simulink subsystem "PvtSubSys_LONC"  (R2020b)
settings: Solver=VariableStepAuto  StartTime=0.0  StopTime=10.0  RelTol=1e-3
undefined symbols (not defined in the file): P_Global_TireRadius_m, P_Global_Weight_N, P_LongCtrl_AxvRoadSlopeThrd, P_LongCtrl_SlideFlagEnable, P_LongCtrl_TotWheelTrqRatio, P_LongCtrl_VLC_fRollCoef, P_LongCtrl_VLC_WindArea, P_LongCtrl_VLCaccelMinHoldXAxis, P_LongCtrl_VLCaccelMinHoldYAxis, P_LongCtrl_VLCaccelMinSlidHoldXAxis, P_LongCtrl_VLCaccelMinSlidHoldYAxis, P_LongCtrl_VLCaDiffCharCoefKiEnableXAxis, P_LongCtrl_VLCaDiffCharCoefKiXAxis, P_LongCtrl_VLCaDtThresUpdateTorq, P_LongCtrl_VLCaXCDeadZoneProp_Y, P_LongCtrl_VLCaxCtrlDevDeadZoneChar_Y, P_LongCtrl_VLCaxCtrlDevEC2DCMax, P_LongCtrl_VLCaxCtrlDevFastQuitDCMode, P_LongCtrl_VLCaxCtrlDevThresAddEC2DCCharYAxis, P_LongCtrl_VLCaxCtrlDevTresAddDC2ECYAxis, P_LongCtrl_VLCaxDtCharAxCtrlDevTresAddDC2ECXAxis, P_LongCtrl_VLCaxDtCharAxCtrlDevTresAddEC2DCXAxis, P_LongCtrl_VLCAxTarDtThreEnableI, P_LongCtrl_VLCaxvRoadSlopeDC4CharXAxis, P_LongCtrl_VLCaxvRoadSlopeDC4CharYAxis, P_LongCtrl_VLCAxvTracMinDC1FullFillXAxis, P_LongCtrl_VLCAxvTracMinDC1FullFillYAxis, P_LongCtrl_VLCcoefFXAxis, P_LongCtrl_VLCcoefFYAxis, P_LongCtrl_VLCcoefIFadeOut1Calc, P_LongCtrl_VLCcoefIFadeOut1Condition, P_LongCtrl_VLCcoefIFadeOut2Calc, P_LongCtrl_VLCcoefIFadeOut2Condition, P_LongCtrl_VLCcoefIFadeOut3Calc, P_LongCtrl_VLCcoefIFadeOut3Condition, P_LongCtrl_VLCcoefKiDiffDtEnlargeYAxis, P_LongCtrl_VLCcoefKiEnableYAxis, P_LongCtrl_VLCcoefKiEnlargeADiffYAxis, P_LongCtrl_VLCcoefPIYAxis, P_LongCtrl_VLCCounterAxvTracMinTimeout, P_LongCtrl_VLCCounterDC2ECTorqDelay, P_LongCtrl_VLCCounterDrvOff2EC, P_LongCtrl_VLCdaxTarEC2DCMax, P_LongCtrl_VLCdiffDtCharCoefKiEnlargeXAxis, P_LongCtrl_VLCdriveOffAxUpLimXAxix, P_LongCtrl_VLCdriveOffAxUpLimYAxix, P_LongCtrl_VLCDtAxvRef2UpperBandDC5, P_LongCtrl_VLCengEfficientCharYAxis, P_LongCtrl_VLCengInverseEfficientYAxis, P_LongCtrl_VLCIACompensionNeg, P_LongCtrl_VLCIACompensionPos, P_LongCtrl_VLCjerkHoldXAxis, P_LongCtrl_VLCjerkHoldYAxis, P_LongCtrl_VLCjerkSlidHoldXAxis, P_LongCtrl_VLCjerkSlidHoldYAxis, P_LongCtrl_VLCki, P_LongCtrl_VLCkp, P_LongCtrl_VLCks, P_LongCtrl_VLCLowerJerkCounterDrvOff2EC, P_LongCtrl_VLCMaRatioCharMaYAxis ... (+12)
libraries: simulink x34
(part 1 of 3)
settings Model: Creator=GW00133806  LastModifiedBy=GW00201118

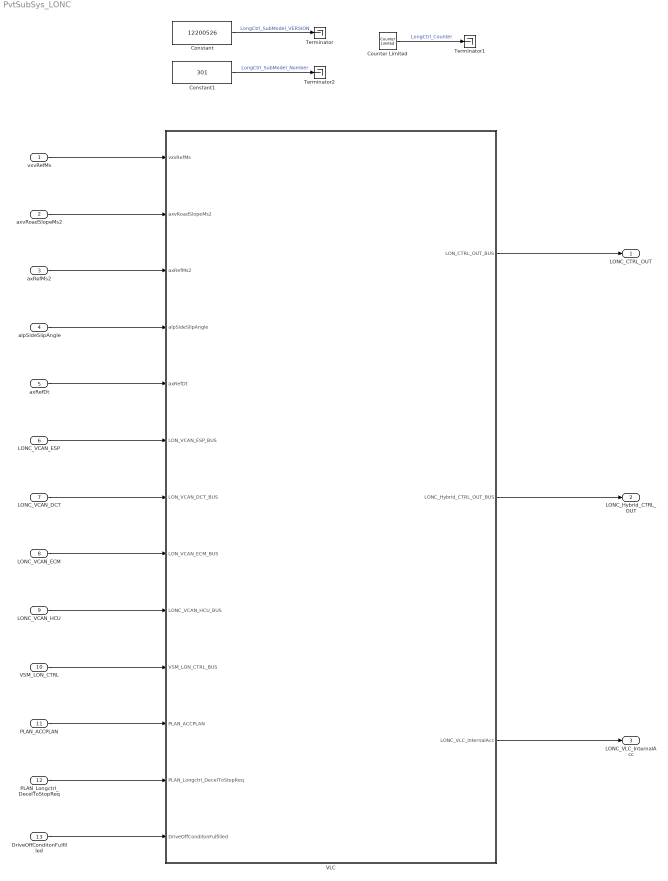
== system PvtSubSys_LONC ==
  vxvRefMs : Inport  Description=m/s | 车速  OutDataTypeStr=single  PortDimensions=1  BusOutputAsStruct=on
  axvRoadSlopeMs2 : Inport  Description=m/s^2 | 坡道加速度  Port=2  OutDataTypeStr=single  PortDimensions=1  BusOutputAsStruct=on
  axRefMs2 : Inport  Description=m/s^2 | 自车参考加速度  Port=3  OutDataTypeStr=single  PortDimensions=1  BusOutputAsStruct=on
  alpSideSlipAngle : Inport  Description=rad | 后轮侧滑角  Port=4  OutDataTypeStr=single  PortDimensions=1  BusOutputAsStruct=on
  axRefDt : Inport  Description=m/s^3 | 加速度变化率  Port=5  OutDataTypeStr=single  PortDimensions=1  BusOutputAsStruct=on
  LONC_VCAN_ESP : Inport  Description=|  Port=6  OutDataTypeStr=Bus: VCAN_ESP_MSG_BUS  PortDimensions=1  BusOutputAsStruct=on
      | NoBrkForce          是否存在轮缸压力
      | VehStandstill       判断车辆是否静止
  LONC_VCAN_DCT : Inport  Description="SHIFT_IN_PROGRESS    换挡进行中"  Port=7  OutDataTypeStr=Bus: VCAN_DCT_MSG_BUS  PortDimensions=1  BusOutputAsStruct=on
  LONC_VCAN_ECM : Inport  Description=|  Port=8  OutDataTypeStr=Bus: VCAN_ECM_MSG_BUS  PortDimensions=1  BusOutputAsStruct=on
      | NetEngTrq               当前实际扭矩
      | MaxEngTrqNorm           最大扭矩
      | EngTrqMinAct            最小可执行扭矩
      | EngTrqMaxActSpd
      | EngSpd                  发动机转速
  LONC_VCAN_HCU : Inport  Port=9  OutDataTypeStr=Bus: VCAN_HCU_MSG_BUS  PortDimensions=1  BusOutputAsStruct=on
  VSM_LON_CTRL : Inport  Description=|  Port=10  OutDataTypeStr=Bus: VSM_LON_CTRL_BUS  PortDimensions=1  BusOutputAsStruct=on
      | ACCSts              ACC状态
      | ACC_DrvOffReq       起步标志位
  PLAN_ACCPLAN : Inport  Description=|  Port=11  OutDataTypeStr=Bus: PLAN_ACCPLAN_BUS
      | ACC_axvCvAim                         期望加速度
      | ACC_axv_ComfortBandLowerValue        期望加速度下限
      | ACC_axv_ComfortBandUpperValue        期望加速度上限
      | ACC_DecelerateJerk                   加速度变化率下限
      | ACC_AccelerateJerk                   加速度变化率上限
      | ACC_BrakePrefer                      制动优先标志位
  PLAN_Longctrl_DecelToStopReq : Inport  Description=boolean | 制动到停状态  Port=12  OutDataTypeStr=boolean  PortDimensions=1  BusOutputAsStruct=on
  DriveOffConditonFulfilled : Inport  Port=13
  Constant : Constant  Value=12200526  OutDataTypeStr=uint32
  Constant1 : Constant  Value=301  OutDataTypeStr=uint32
  Counter Limited : simulink/Sources/Counter Limited  uplimit=15  tsamp=-1
  Terminator : Terminator
  Terminator1 : Terminator
  Terminator2 : Terminator
  VLC : Subsystem
  LONC_CTRL_OUT : Outport  OutDataTypeStr=Bus: LONC_CTRL_OUT_BUS  PortDimensions=1  BusOutputAsStruct=on
  LONC_Hybrid_CTRL_OUT : Outport  Port=2  OutDataTypeStr=Bus: LONC_Hybrid_CTRL_OUT_BUS  PortDimensions=1  BusOutputAsStruct=on
  LONC_VLC_InternalAcc : Outport  Port=3  OutDataTypeStr=single
  wires:
  vxvRefMs/1 -> VLC/1(vxvRefMs)
  LONC_VCAN_ECM/1 -> VLC/8(LON_VCAN_ECM_BUS)
  Counter Limited/1 -> Terminator1/1  "LongCtrl_Counter"
  Constant/1 -> Terminator/1  "LongCtrl_SubModel_VERSION"
  DriveOffConditonFulfilled/1 -> VLC/13(DriveOffConditonFulfilled)
  VSM_LON_CTRL/1 -> VLC/10(VSM_LON_CTRL_BUS)
  axRefMs2/1 -> VLC/3(axRefMs2)
  alpSideSlipAngle/1 -> VLC/4(alpSideSlipAngle)
  PLAN_Longctrl_DecelToStopReq/1 -> VLC/12(PLAN_Longctrl_DecelToStopReq)
  LONC_VCAN_DCT/1 -> VLC/7(LON_VCAN_DCT_BUS)
  axvRoadSlopeMs2/1 -> VLC/2(axvRoadSlopeMs2)
  VLC/3(LONC_VLC_InternalAcc) -> LONC_VLC_InternalAcc/1
  axRefDt/1 -> VLC/5(axRefDt)
  LONC_VCAN_HCU/1 -> VLC/9(LONC_VCAN_HCU_BUS)
  VLC/1(LON_CTRL_OUT_BUS) -> LONC_CTRL_OUT/1
  PLAN_ACCPLAN/1 -> VLC/11(PLAN_ACCPLAN)
  LONC_VCAN_ESP/1 -> VLC/6(LON_VCAN_ESP_BUS)
  Constant1/1 -> Terminator2/1  "LongCtrl_SubModel_Number"
  VLC/2(LONC_Hybrid_CTRL_OUT_BUS) -> LONC_Hybrid_CTRL_OUT/1

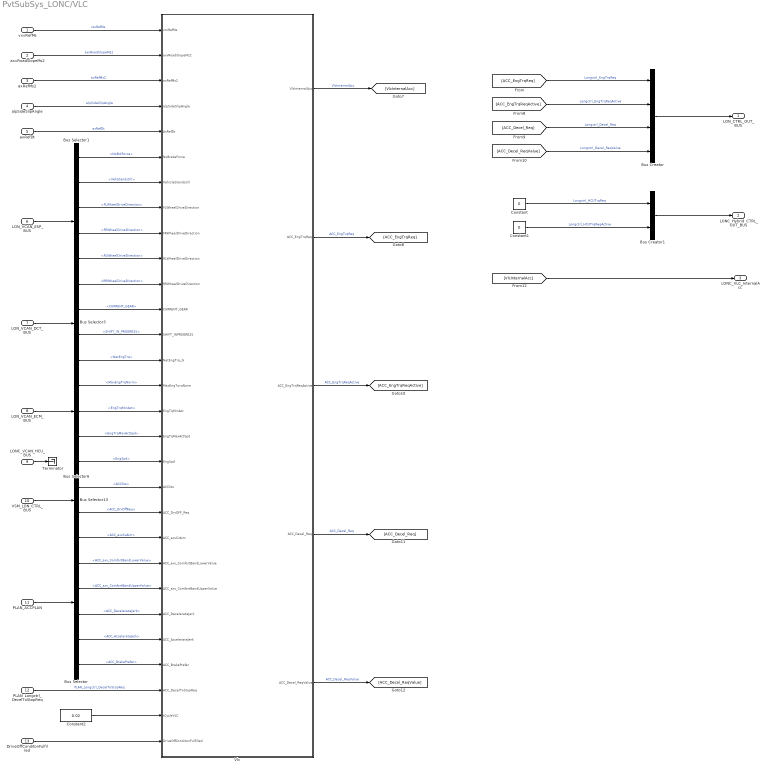
== system PvtSubSys_LONC/VLC ==
  vxvRefMs : Inport
  axvRoadSlopeMs2 : Inport  Port=2
  axRefMs2 : Inport  Port=3
  alpSideSlipAngle : Inport  Port=4
  axRefDt : Inport  Port=5
  LON_VCAN_ESP_BUS : Inport  Port=6  OutDataTypeStr=Bus: VCAN_ESP_MSG_BUS
  LON_VCAN_DCT_BUS : Inport  Port=7  OutDataTypeStr=Bus: VCAN_DCT_MSG_BUS
  LON_VCAN_ECM_BUS : Inport  Port=8  OutDataTypeStr=Bus: VCAN_ECM_MSG_BUS
  LONC_VCAN_HCU_BUS : Inport  Port=9  OutDataTypeStr=Bus: VCAN_HCU_MSG_BUS
  VSM_LON_CTRL_BUS : Inport  Port=10  OutDataTypeStr=Bus: VSM_LON_CTRL_BUS
  PLAN_ACCPLAN : Inport  Port=11  OutDataTypeStr=Bus: PLAN_ACCPLAN_BUS
  PLAN_Longctrl_DecelToStopReq : Inport  Port=12  OutDataTypeStr=boolean
  DriveOffConditonFulfilled : Inport  Port=13
  Bus Creator : BusCreator  Inputs=4  OutDataTypeStr=Bus: LONC_CTRL_OUT_BUS  NonVirtualBus=on
  Bus Creator1 : BusCreator  Inputs=2  OutDataTypeStr=Bus: LONC_Hybrid_CTRL_OUT_BUS  NonVirtualBus=on
  Bus Selector : BusSelector  OutputSignals=ACC_axvCvAim,ACC_axv_ComfortBandLowerValue,ACC_axv_ComfortBandUpperValue,ACC_DecelerateJerk,ACC_AccelerateJerk,ACC_BrakePrefer
  Bus Selector1 : BusSelector  OutputSignals=NoBrkForce,VehStandstill,FLWheelDriveDirection,FRWheelDriveDirection,RLWheelDriveDirection,RRWheelDriveDirection
  Bus Selector13 : BusSelector  OutputSignals=ACCSts,ACC_DrvOffReq
  Bus Selector3 : BusSelector  OutputSignals=CURRENT_GEAR,SHIFT_IN_PROGRESS
  Bus Selector6 : BusSelector  OutputSignals=NetEngTrq,MaxEngTrqNorm,EngTrqMinAct,EngTrqMaxActSpd,EngSpd
  Constant : Constant  Value=0  OutDataTypeStr=single
  Constant1 : Constant  Value=0  OutDataTypeStr=boolean
  Constant2 : Constant  Value=0.02  OutDataTypeStr=single
  Terminator : Terminator
  Vlc : Subsystem  TreatAsAtomicUnit=on
  LON_CTRL_OUT_BUS : Outport  OutDataTypeStr=Bus: LONC_CTRL_OUT_BUS
  LONC_Hybrid_CTRL_OUT_BUS : Outport  Port=2  OutDataTypeStr=Bus: LONC_Hybrid_CTRL_OUT_BUS
  LONC_VLC_InternalAcc : Outport  Port=3  OutDataTypeStr=single
  wires:
  LONC_VCAN_HCU_BUS/1 -> Terminator/1
  Constant/1 -> Bus Creator1/1  "Longctrl_HCUTrqReq"
  Constant1/1 -> Bus Creator1/2  "Longctrl_HCUTrqReqActive"
  Bus Creator1/1 -> LONC_Hybrid_CTRL_OUT_BUS/1
  PLAN_Longctrl_DecelToStopReq/1 -> Vlc/27(ACC_DecelToStopReq)  "PLAN_Longctrl_DecelToStopReq"
  [VlcInternalAcc] -> LONC_VLC_InternalAcc/1
  Bus Selector/1 -> Vlc/21(ACC_axvCvAim)  "<ACC_axvCvAim>"
  Bus Selector/6 -> Vlc/26(ACC_BrakePrefer)  "<ACC_BrakePrefer>"
  Bus Selector/2 -> Vlc/22(ACC_axv_ComfortBandLowerValue)  "<ACC_axv_ComfortBandLowerValue>"
  Bus Selector/3 -> Vlc/23(ACC_axv_ComfortBandUpperValue)  "<ACC_axv_ComfortBandUpperValue>"
  Bus Selector/5 -> Vlc/25(ACC_AccelerateJerk)  "<ACC_AccelerateJerk>"
  Bus Selector/4 -> Vlc/24(ACC_DecelerateJerk)  "<ACC_DecelerateJerk>"
  PLAN_ACCPLAN/1 -> Bus Selector/1
  alpSideSlipAngle/1 -> Vlc/4(alpSideSlipAngle)  "alpSideSlipAngle"
  Bus Selector13/2 -> Vlc/20(ACC_DrvOFF_Req)  "<ACC_DrvOffReq>"
  Bus Selector13/1 -> Vlc/19(ACCSts)  "<ACCSts>"
  VSM_LON_CTRL_BUS/1 -> Bus Selector13/1
  Bus Selector6/5 -> Vlc/18(EngSpd)  "<EngSpd>"
  Bus Selector6/4 -> Vlc/17(EngTqMaxActSpd)  "<EngTrqMaxActSpd>"
  Bus Selector6/3 -> Vlc/16(EngTqMinAct)  "<EngTrqMinAct>"
  Bus Selector6/2 -> Vlc/15(MaxEngTorqNorm)  "<MaxEngTrqNorm>"
  Bus Selector6/1 -> Vlc/14(NetEngTrq_G)  "<NetEngTrq>"
  LON_VCAN_ECM_BUS/1 -> Bus Selector6/1
  LON_VCAN_DCT_BUS/1 -> Bus Selector3/1
  Bus Selector3/2 -> Vlc/13(SHIFT_INPROGRESS)  "<SHIFT_IN_PROGRESS>"
  Bus Selector3/1 -> Vlc/12(CURRENT_GEAR)  "<CURRENT_GEAR>"
  LON_VCAN_ESP_BUS/1 -> Bus Selector1/1
  Bus Selector1/2 -> Vlc/7(VehicleStandstill)  "<VehStandstill>"
  Bus Selector1/1 -> Vlc/6(NoBrakeForce)  "<NoBrkForce>"
  axRefDt/1 -> Vlc/5(AxRefDt)  "axRefDt"
  axRefMs2/1 -> Vlc/3(axRefMs2)  "axRefMs2"
  axvRoadSlopeMs2/1 -> Vlc/2(axvRoadSlopeMs2)  "axvRoadSlopeMs2"
  vxvRefMs/1 -> Vlc/1(vxvRefMs)  "vxvRefMs"
  [ACC_EngTrqReqActive] -> Bus Creator/2  "Longctrl_EngTrqReqActive"
  Vlc/2(ACC_EngTrqReq) -> [ACC_EngTrqReq]  "ACC_EngTrqReq"
  Vlc/4(ACC_Decel_Req) -> [ACC_Decel_Req]  "ACC_Decel_Req"
  Vlc/1(VlcInternalAcc) -> [VlcInternalAcc]  "VlcInternalAcc"
  Vlc/5(ACC_Decel_ReqValue) -> [ACC_Decel_ReqValue]  "ACC_Decel_ReqValue"
  Vlc/3(ACC_EngTrqReqActive) -> [ACC_EngTrqReqActive]  "ACC_EngTrqReqActive"
  Bus Creator/1 -> LON_CTRL_OUT_BUS/1
  [ACC_Decel_Req] -> Bus Creator/3  "Longctrl_Decel_Req"
  [ACC_Decel_ReqValue] -> Bus Creator/4  "Longctrl_Decel_ReqValue"
  [ACC_EngTrqReq] -> Bus Creator/1  "Longctrl_EngTrqReq"
  Constant2/1 -> Vlc/28(tCycleVLC)
  DriveOffConditonFulfilled/1 -> Vlc/29(DriveOffConditonFulfilled)
  Bus Selector1/3 -> Vlc/8(FLWheelDriveDirection)  "<FLWheelDriveDirection>"
  Bus Selector1/4 -> Vlc/9(FRWheelDriveDirection)  "<FRWheelDriveDirection>"
  Bus Selector1/5 -> Vlc/10(RLWheelDriveDirection)  "<RLWheelDriveDirection>"
  Bus Selector1/6 -> Vlc/11(RRWheelDriveDirection)  "<RRWheelDriveDirection>"

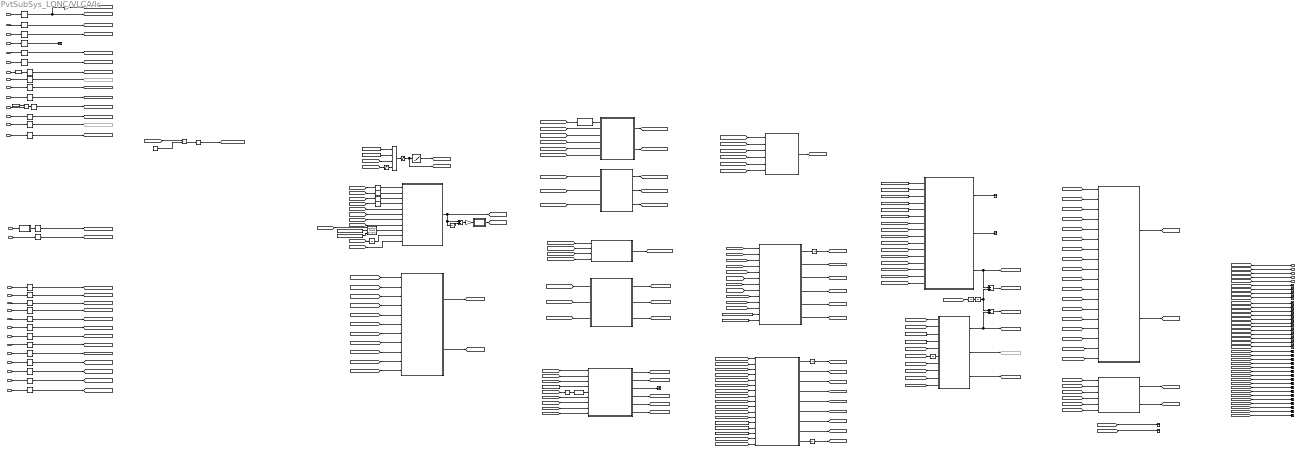
== system PvtSubSys_LONC/VLC/Vlc ==
  vxvRefMs : Inport  OutDataTypeStr=single
  axvRoadSlopeMs2 : Inport  Port=2  OutDataTypeStr=single
  axRefMs2 : Inport  Port=3  OutDataTypeStr=single
  alpSideSlipAngle : Inport  Port=4  OutDataTypeStr=single
  AxRefDt : Inport  Port=5  OutDataTypeStr=single
  NoBrakeForce : Inport  Port=6  OutDataTypeStr=boolean
  VehicleStandstill : Inport  Port=7  OutDataTypeStr=uint8
  FLWheelDriveDirection : Inport  Port=8
  FRWheelDriveDirection : Inport  Port=9
  RLWheelDriveDirection : Inport  Port=10
  RRWheelDriveDirection : Inport  Port=11
  CURRENT_GEAR : Inport  Port=12  OutDataTypeStr=uint8
  SHIFT_INPROGRESS : Inport  Port=13  OutDataTypeStr=boolean
  NetEngTrq_G : Inport  Port=14  OutDataTypeStr=single
  MaxEngTorqNorm : Inport  Port=15  OutDataTypeStr=uint16
  EngTqMinAct : Inport  Port=16  OutDataTypeStr=single
  EngTqMaxActSpd : Inport  Port=17  OutDataTypeStr=single
  EngSpd : Inport  Port=18  OutDataTypeStr=single
  ACCSts : Inport  Port=19  OutDataTypeStr=uint8
  ACC_DrvOFF_Req : Inport  Port=20  OutDataTypeStr=boolean
  ACC_axvCvAim : Inport  Port=21
  ACC_axv_ComfortBandLowerValue : Inport  Port=22
  ACC_axv_ComfortBandUpperValue : Inport  Port=23
  ACC_DecelerateJerk : Inport  Port=24
  ACC_AccelerateJerk : Inport  Port=25
  ACC_BrakePrefer : Inport  Port=26
  ACC_DecelToStopReq : Inport  Port=27
  tCycleVLC : Inport  Port=28
  DriveOffConditonFulfilled : Inport  Port=29
  AxTarUplimit : simulink/Lookup Tables/Lookup Table Dynamic  LookUpMeth=Interpolation-Use End Values  OutDataType=fixdt('single')  OutScaling=[]  OutputDataTypeScalingMode=Specify via dialog  OutDataTypeStr=single  DoSatur=off
  Compare To Constant8 : simulink/Logic and Bit Operations/Compare To Constant  relop===  const=1  OutDataTypeStr=boolean
  Compare To Zero : simulink/Logic and Bit Operations/Compare To Zero  relop===  OutDataTypeStr=boolean
  Constant : Constant  OutDataTypeStr=single
  Constant1 : Constant  Description="1.5         1.5         1.6         1.8           2"  Value=P_LongCtrl_VLCdriveOffAxUpLimYAxix  OutDataTypeStr=single
      settings: AttributesFormatString=%<Description>
  Constant10 : Constant  Description=0.7  Value=P_LongCtrl_VLCaxCtrlDevFastQuitDCMode  OutDataTypeStr=single
      settings: AttributesFormatString=%<Description>
  Constant11 : Constant  Description="0.1         0.1        0.15         0.2         0.2"  Value=P_LongCtrl_VLCaxCtrlDevThresAddEC2DCCharYAxis  OutDataTypeStr=single
      settings: AttributesFormatString=%<Description>
  Constant12 : Constant  Description=0.5  Value=P_LongCtrl_VLCaxCtrlDevEC2DCMax  OutDataTypeStr=single
      settings: AttributesFormatString=%<Description>
  Constant13 : Constant  Description=-0.2  Value=P_LongCtrl_VLCdaxTarEC2DCMax  OutDataTypeStr=single
      settings: AttributesFormatString=%<Description>
  Constant2 : Constant  Description=4  Value=P_LongCtrl_VLCkp  OutDataTypeStr=single
      settings: AttributesFormatString=%<Description>
  Constant3 : Constant  Description="0         0.5           1         1.5           3"  Value=P_LongCtrl_VLCdriveOffAxUpLimXAxix  OutDataTypeStr=single
      settings: AttributesFormatString=%<Description>
  Constant4 : Constant  Description=0.05  Value=P_LongCtrl_VLCki  OutDataTypeStr=single
      settings: AttributesFormatString=%<Description>
  Constant5 : Constant  Description="60  10   0   0   0  10  60"  Value=P_LongCtrl_VLCaXCDeadZoneProp_Y  OutDataTypeStr=single
      settings: AttributesFormatString=%<Description>
  Constant8 : Constant  Value=10  OutDataTypeStr=single
  Constant9 : Constant  Description="0.15        0.15        0.12         0.1         0.1"  Value=P_LongCtrl_VLCaxCtrlDevTresAddDC2ECYAxis  OutDataTypeStr=single
      settings: AttributesFormatString=%<Description>
  DC : Subsystem
  Data Type Conversion : DataTypeConversion  OutDataTypeStr=single
  EC : Subsystem
  FF_Control : Subsystem
  FxvCompensate : Constant  Value=0  OutDataTypeStr=single
  Gain1 : Gain  Gain=3.6  ParamDataTypeStr=single
  Gain2 : Gain  Gain=50
  Goto : Goto  Commented=on  GotoTag=CAN_Gear
  Goto26 : Goto  Commented=on  GotoTag=FFShiftInput
  Goto8 : Goto  Commented=on  GotoTag=CAN_EngTqMaxAct
  Ks : Constant  Description=0.45  Value=P_LongCtrl_VLCks  OutDataTypeStr=single
      settings: AttributesFormatString=%<Description>
  LP : Subsystem
  LP1 : Subsystem
  Ma_Ratio : Lookup_n-D  NumberOfTableDimensions=1  BreakpointsForDimension1=P_LongCtrl_VLCTrRatioCharMaXAxis  Table=P_LongCtrl_VLCMaRatioCharMaYAxis  ExtrapMethod=Clip  UseLastTableValue=on  RndMeth=Simplest  InputSameDT=on
  MinMax1 : MinMax  Function=max  Inputs=2  OutDataTypeStr=single
  PI_Control : Subsystem
  PVLCaXCKiCtrlDevChar_Y : Constant  Description="1           1         0.9        0.85         0.7         0.6         0.7        0.85         0.9           1           1"  Value=P_LongCtrl_VLCcoefKiEnlargeADiffYAxis  OutDataTypeStr=single
      settings: AttributesFormatString=%<Description>
  P_VlcAxCtrlDevDeadZoneChar_Y : Constant  Description="0.15        0.15        0.18         0.2         0.2"  Value=P_LongCtrl_VLCaxCtrlDevDeadZoneChar_Y  OutDataTypeStr=single
      settings: AttributesFormatString=%<Description>
  Product : Product  OutDataTypeStr=single
  Product5 : Product  Inputs=***/  RndMeth=Zero
  Saturation1 : Saturate  UpperLimit=180  LowerLimit=1.08
  Saturation2 : Saturate  UpperLimit=P_LongCtrl_VLCTrTatioMax  LowerLimit=P_LongCtrl_VLCTrTatioMin
  Signal Copy{,1..28} (29 alike) : SignalConversion  OverrideOpt=off
  SlidJudge : Subsystem
  Subsystem : Subsystem
  Sum1 : Sum
  Sum2 : Sum
  Sum8 : Sum  Inputs=+-
  SwitchToBrakeMode : Subsystem
  SwitchToDriveMode : Subsystem
  Tapped Delay{2..5} (4 alike) : simulink/Discrete/Tapped Delay  vinit=0.0  samptime=-1  NumDelays=1  DelayOrder=Newest  includeCurrent=on
  Terminator{,1,3..23,25..37,45..46,48} (39 alike) : Terminator
  Trigonometric Function : Trigonometry  Operator=asin
  Unit Delay{,1..7} (8 alike) : UnitDelay  SampleTime=-1  HasFrameUpgradeWarning=on
  UpdateFlagCalc : Subsystem
  VLC_control_sts : Stateflow chart  TreatAsAtomicUnit=on
  VlcInternalAccCalc : MATLAB Function  TreatAsAtomicUnit=on
  VlcInternalFail : Constant  Value=0  OutDataTypeStr=uint8
  Weight/N1 : Constant  Value=0.377  OutDataTypeStr=single
  Weight/N2 : Constant  Value=P_Global_TireRadius_m
  axvClosedLoopControlCalc : Subsystem
  axvModelResidualCalc : Subsystem
  axvTracActMean_calc : Subsystem
  axvTracMin_calc : Subsystem
  g : Constant  Value=1/10  OutDataTypeStr=single
  VlcInternalAcc : Outport
  ACC_EngTrqReq : Outport  Port=2
  ACC_EngTrqReqActive : Outport  Port=3
  ACC_Decel_Req : Outport  Port=4
  ACC_Decel_ReqValue : Outport  Port=5
  wires:
  ACCSts/1 -> Subsystem/1(u)  "ACCSts"
  [ACC_DecelToStopReq] -> SwitchToDriveMode/11(StopReq)
  [VehSts_axvRoadSlope] -> DC/4(axvRoadSlopeMs2)
  SwitchToBrakeMode/4(Swit2DC_3) -> [SwDC_3]
  [VehSts_axvRoadSlope] -> SwitchToBrakeMode/4(axvRoadSlope)
  [CAN_ShiftInProgress] -> SwitchToBrakeMode/9("ShiftInProgress ")
  Constant12/1 -> SwitchToBrakeMode/14(P_VlcAxCtrlDevEC2DCMax)
  [AxRef_ms2] -> SwitchToBrakeMode/11(axRef)
  [ACCSts_ACCModeSts] -> SwitchToBrakeMode/7(ACC_Mode)
  [ACC_DecelToStopReq] -> SwitchToBrakeMode/6(StopReq)
  Unit Delay6/1 -> [SwDC]
  SwitchToBrakeMode/6(Swit2DC_5) -> [SwDC_5]
  [axvTracMin] -> SwitchToBrakeMode/2(axvTracMin)
  SwitchToBrakeMode/9(Override2DC) -> Unit Delay2/1
  [ACC_BrakePrefer] -> SwitchToBrakeMode/10(BrakePrefer)
  SwitchToBrakeMode/3(Swit2DC_2) -> [SwDC_2]
  Constant11/1 -> SwitchToBrakeMode/13(P_LongCtrl_VLCAxCtrlDevTresAddEC2DC)
  SwitchToBrakeMode/2(Swit2DC_1) -> [SwDC_1]
  SwitchToBrakeMode/1(SwitchToBrakeMode) -> Unit Delay6/1
  SwitchToBrakeMode/5(Swit2DC_4) -> [SwDC_4]
  [VlcAxTarDt] -> SwitchToBrakeMode/12(VlcAxTarDt)
  [VlcInternalAcc] -> SwitchToBrakeMode/5(VlcAxTar)
  Unit Delay2/1 -> [OverrideToDC]
  [ACC_axvCvAim] -> SwitchToBrakeMode/3(axvCvAim)
  [ACC_axvComfortBandUpperValue] -> SwitchToBrakeMode/8(axv_ComfortBandUpperValue)
  SwitchToBrakeMode/7(Swit2DC_6) -> [SwDC_6]
  [VehSts_VxvRef_ms] -> SwitchToBrakeMode/1(VxvRef_ms)
  [CAN_NetEngTrq] -> SwitchToBrakeMode/17(CAN_NetEngTrq)
  [ACC_EngTorqReq] -> SwitchToBrakeMode/16(ACC_EngTorqReq)
  SwitchToBrakeMode/8(Swit2DC_7) -> [SwDC_7]
  Constant13/1 -> SwitchToBrakeMode/15(P_VlcdAxTarEC2DCMax)
  Tapped Delay3/1 -> VlcInternalAccCalc/2(DC)
  Tapped Delay5/1 -> VlcInternalAccCalc/4(ACC_Mode)
  [UpdateEnable_axvModeldiff] -> Terminator37/1  "LongCtrl_UpdateEnable_axvModeldiff"
  [FF_NetEngTorqMax] -> Terminator31/1  "LongCtrl_FF_NetEngTorqMax"
  alpSideSlipAngle/1 -> Signal Copy3/1
  Trigonometric Function/1 -> [VehSts_SlopeAngle_rad]
  g/1 -> Product/2
  [VehSts_axvRoadSlope] -> Product/1
  axRefMs2/1 -> Signal Copy2/1
  Unit Delay1/1 -> VlcInternalAccCalc/10(VlcInternalAccK1)
  AxTarUplimit/1 -> VlcInternalAccCalc/9(DriveOffAxUpLim)
  PI_Control/3(PI_NetEngTorq) -> [PI_NetEngTorqInc], Sum1/1  "PI_NetEngTorq"
  [axvClosedLoopControl] -> FF_Control/1(AxTar)
  [Ma_Ratio] -> axvTracMin_calc/5(Ma)
  [PI_NetEngTorqInc] -> EC/14(PI_NetEngTorqInc)
  [ACCSts_ACCModeSts] -> VLC_control_sts/3(ACC_Mode)
  [VehSts_VxvRef_ms] -> AxTarUplimit/1
  [VehSts_VxvRef_kmh] -> axvTracMin_calc/3(VehicleSpd_kmh)
  Saturation1/1 -> Product5/4
  SwitchToDriveMode/1(SwitchToDriveMode) -> Unit Delay7/1
  axvClosedLoopControlCalc/2(tauFxvCvFilter) -> [tauFxvCvFilter]
  [CAN_NetEngTrq] -> LP1/1(Raw)
  [VehSts_VxvRef_ms] -> FF_Control/5(VxvRef_ms)
  [ACC_axvComfortBandLowerValue] -> SwitchToDriveMode/9(axv_ComfortBandLowerValue)
  [CAN_NoBrakeForce] -> UpdateFlagCalc/1(NoBrakeForce)
  [CAN_MaxEngTrq] -> axvTracActMean_calc/2(MaxEngTorq)
  [CAN_EngSpd] -> Product5/3
  Weight/N2/1 -> Product5/2
  Constant9/1 -> SwitchToDriveMode/12(P_VlcAxCtrlDevTresAddDC2EC)
  EC/2(Signal_ACC_EngTrqReqActive) -> [ACC_EngTorqReqActive]  "Signal_ACC_EngTrqReqActive"
  axvClosedLoopControlCalc/1(axvClosedLoopControl) -> [axvClosedLoopControl]
  [ACC_UpperJerk] -> EC/4(Accelerate_jerk)
  [ECEnable] -> PI_Control/10(ECEnable)
  [VehSts_VxvRef_kmh] -> PI_Control/9(Vego_kmh)
  [Tr_Ratio] -> axvTracActMean_calc/6(Tr)
  [CAN_ShiftInProgress] -> EC/11(ShiftInProgress)
  [CAN_ShiftInProgress] -> UpdateFlagCalc/2(DCT_ShiftInProgress)
  [tauFxvCvFilter] -> FF_Control/10(tauFxvCvFilter)
  [UpdateEnable_axvModeldiff] -> axvModelResidualCalc/2(Enable)
  [Tr_Ratio] -> axvTracMin_calc/6(Tr)
  PI_Control/1(Diff_grad) -> Terminator45/1
  [CAN_MaxEngTrq] -> axvTracMin_calc/2(MaxEngTorq)
  [Ma_Ratio] -> axvTracActMean_calc/5(Ma)
  VLC_control_sts/2(tEC) -> [tEC]
  [ACCSts_ACCModeSts] -> DC/3(ACCmode)
  [Tr_Ratio] -> FF_Control/8(Tr_Ratio)
  [ACC_BrakePrefer] -> SwitchToDriveMode/10(BrakePrefer)
  EC/1(ACC_EngTorqReq) -> [ACC_EngTorqReq]  "Signal_ACC_EngTrqReq"
  Unit Delay3/1 -> Unit Delay4/1
  Constant3/1 -> AxTarUplimit/2
  Weight/N1/1 -> Product5/1
  [ACC_axvCvAim] -> SwitchToDriveMode/8(AxvCvAim)
  [VlcInternalAcc] -> axvClosedLoopControlCalc/2(VlcInternalAcc)
  [VehSts_VxvRef_ms] -> EC/5(VxvRef_ms)
  Constant2/1 -> PI_Control/1(P_Gain)
  [axvDiff] -> PI_Control/8(axvDiff)
  [ACC_LowerJerk] -> EC/6(Decelerate_jerk)
  [AxRef_ms2] -> axvClosedLoopControlCalc/3(AxRef)
  [axvModelResidual] -> axvClosedLoopControlCalc/1(axvModelResidual)
  [ACC_LowerJerk] -> VlcInternalAccCalc/8(DeceJerk)
  [ACCSts_ACCModeSts] -> Tapped Delay5/1
  Compare To Zero/1 -> Data Type Conversion/1
  Sum8/1 -> Gain2/1
  axvClosedLoopControlCalc/3(Diff) -> [axvDiff]
  [FF_EngTorqInc] -> EC/13(FF_EngTorqInc)
  [AxRef_ms2] -> PI_Control/13(axvRef)
  [VlcInternalAcc] -> Unit Delay1/1
  Unit Delay4/1 -> Sum1/2, Sum2/1
  VlcInternalAccCalc/1(VlcInternalAcc) -> [VlcInternalAcc], Unit Delay5/1, Sum8/1
  [VehSts_SlopeAngle_rad] -> axvTracActMean_calc/4(SlopeAngle_rad)
  [VehSts_VxvRef_kmh] -> axvTracActMean_calc/3(VehicleSpd_kmh)
  [tEC] -> EC/3(tEC)
  UpdateFlagCalc/1(UpdateEnable) -> [UpdateEnable_axvModeldiff]
  VLC_control_sts/3(tDC) -> Terminator/1
  SwitchToDriveMode/6(Swit2EC_5) -> [SwEC_5]
  LP1/1(Out) -> axvTracActMean_calc/1(Torq)
  [CAN_MaxEngTrq] -> EC/10(MaxEngTrq)
  LP/1(Out) -> [VlcAxTarDt]
  axvTracActMean_calc/1(axvTracActMean) -> [axvTracActMean]
  [CAN_MaxEngTrq] -> FF_Control/7(MaxEngTrq)
  SwitchToDriveMode/4(Swit2EC_3) -> [SwEC_3]
  [ACCSts_DriveOffReq] -> Tapped Delay4/1
  [AxRef_ms2] -> SwitchToDriveMode/5(axRef)
  [CAN_ShiftInProgress] -> PI_Control/15(ShiftInProgress)
  PI_Control/2(BigDeadzoneValue) -> Terminator46/1
  [ACC_axvCvAim] -> VlcInternalAccCalc/6(AxTar)
  axvModelResidualCalc/3(axvModelResidual) -> [axvModelResidual]
  Data Type Conversion/1 -> VLC_control_sts/5(Motorial)
  [CAN_EngSpd] -> EC/2(EngSpd)
  [VehSts_SlopeAngle_rad] -> axvTracMin_calc/4(SlopeAngle_rad)
  [VlcInternalAcc] -> DC/2(VlcAxTar)
  [DCEnable] -> DC/1(DC_enable)
  [AxRef_ms2] -> axvModelResidualCalc/1(AxRef)
  Unit Delay7/1 -> [SwEC]
  [AxRef_ms2] -> VlcInternalAccCalc/5(AxRef)
  Sum2/1 -> [FF_NetEngTorq]
  Ma_Ratio/1 -> [Ma_Ratio]
  Saturation2/1 -> Ma_Ratio/1, [Tr_Ratio]
  [Fz] -> FF_Control/2(Fz)
  Constant5/1 -> PI_Control/3(P_VlcAXCDeadZoneProp_Y)
  Sum1/1 -> [PI_NetEngTorq]
  DC/2(ACC_Decel_ReqValue) -> [ACC_DecelReqValue]  "Signal_ACC_Decel_ReqValue"
  [ACCSts_ACCModeSts] -> SwitchToDriveMode/1(ACC_Mode)
  [SwEC] -> VLC_control_sts/1(SwitchToDriveMode)
  [VlcInternalAcc] -> SwitchToDriveMode/6(VlcAxTar)
  axvTracMin_calc/1(axvTracMin) -> [axvTracMin]
  [ECEnable] -> EC/1(ECEnable)
  VLC_control_sts/4(DCEnable) -> [DCEnable]
  [CAN_MaxEngTrq] -> PI_Control/12(MaxEngTrq)
  [Tr_Ratio] -> PI_Control/11(Tr_Ratio)
  [VehSts_VxvRef_kmh] -> Saturation1/1
  P_VlcAxCtrlDevDeadZoneChar_Y/1 -> PI_Control/4(P_VlcAxCtrlDevDeadZoneChar_Y)
  axvModelResidualCalc/2(axvModel_Ref) -> [axvModelRef]
  FF_Control/3(FF_NetEngTorqMax) -> [FF_NetEngTorqMax]
  FF_Control/1(FF_NetEngTorqInc) -> [FF_EngTorqInc], Sum2/2
  [SwDC] -> VLC_control_sts/2(SwitchToBrakeMode)
  [CAN_EngTqMinAct] -> axvTracMin_calc/1(Torq)
  FF_Control/2(FFShiftInput) -> Goto26/1
  axvTracActMean_calc/2(Fz) -> [Fz]
  [OverrideToDC] -> VLC_control_sts/6(OverrideToDC)
  SwitchToDriveMode/2(Swit2EC_1) -> [SwEC_1]
  Unit Delay/1 -> FF_Control/6(ACC_EngTorqReqK1)
  [CAN_NetEngTrq] -> EC/12(NetEngTrq)
  SwitchToDriveMode/5(Swit2EC_4) -> [SwEC_4]
  Unit Delay5/1 -> Sum8/2
  [ACCSts_VehStandstill] -> Compare To Zero/1
  Tapped Delay2/1 -> VlcInternalAccCalc/1(EC)
  PVLCaXCKiCtrlDevChar_Y/1 -> PI_Control/5(P_LongCtrl_VLCcoefKiEnlargeADiff)
  [ACC_UpperJerk] -> VlcInternalAccCalc/7(AcceJerk)
  VlcInternalFail/1 -> VLC_control_sts/4(VLCInternalFailSts)
  DC/1(ACC_Decel_Req) -> [ACC_DecelReq]  "Signal_ACC_Decel_Req"
  [VehSts_axvRoadSlope] -> SwitchToDriveMode/4(AxvRoadSlope)
  Gain2/1 -> LP/1(Raw)
  [DCEnable] -> Tapped Delay3/1
  axvModelResidualCalc/1(axvModeldiff) -> [axvModeldiff]
  [axvTracActMean] -> axvModelResidualCalc/3(axvTorqMean)
  [CAN_NoBrakeForce] -> SwitchToDriveMode/3(NoBrakeForce)
  [Ma_Ratio] -> EC/8(Ma_Ratio)
  [VlcAxTarDt] -> SwitchToDriveMode/7(VlcAxTarDt)
  [DCEnable] -> EC/7(DCEnable)
  FxvCompensate/1 -> FF_Control/4(FxvCompensate)
  Product5/1 -> Saturation2/1
  SwitchToDriveMode/3(Swit2EC_2) -> [SwEC_2]
  [VlcAxTarDt] -> PI_Control/7(VlcAxTarDt)
  [ACC_EngTorqReq] -> Unit Delay/1
  Constant10/1 -> SwitchToDriveMode/13(P_VlcAxCtrlDevFastQuitDCMode)
  [VlcInternalAcc] -> PI_Control/14(GetVlcAxTar)
  [VehSts_AxRefDt] -> UpdateFlagCalc/3(AxRefDt)
  [VehSts_VxvRef_kmh] -> UpdateFlagCalc/4(Vxv)
  [ACCSts_DriveOffReq] -> EC/15(DiveOff)
  [Ma_Ratio] -> FF_Control/9(Ma_Ratio)
  [CAN_NetEngTrq] -> Unit Delay3/1
  [ECEnable] -> Tapped Delay2/1
  Constant8/1 -> PI_Control/6(P_VlcWindupLim)
  [ACCSts_DriveOffReq] -> SwitchToDriveMode/2(DriveOff)
  Tapped Delay4/1 -> VlcInternalAccCalc/3(DriveOff)
  Ks/1 -> FF_Control/3(Ks_Gain)
  Constant1/1 -> AxTarUplimit/3
  VLC_control_sts/1(ECEnable) -> [ECEnable]
  Constant4/1 -> PI_Control/2(I_Gain)
  [Tr_Ratio] -> EC/9(Tr_Ratio)
  [SwDC_4] -> Terminator21/1  "LongCtrl_Sw2DC4"
  [SwEC] -> Terminator33/1  "LongCtrl_Sw2EC"
  [Fz] -> Terminator9/1  "LongCtrl_Fz"
  [SwDC_5] -> Terminator22/1  "LongCtrl_Sw2DC5"
  [axvModelRef] -> Terminator15/1  "LongCtrl_axvModelRef"
  [SwDC] -> Terminator25/1  "LongCtrl_Sw2DC"
  [ACC_DecelReq] -> ACC_Decel_Req/1  "LongCtrl_ACC_Decel_Req"
  [axvModeldiff] -> Terminator20/1  "LongCtrl_axvModelDiff"
  [axvDiff] -> Terminator17/1  "LongCtrl_axvDiff"
  [OverrideToDC] -> Terminator12/1  "LongCtrl_OverrideToDC"
  [FF_EngTorqInc] -> Terminator8/1  "LongCtrl_FF_NetEngTorqInc"
  [axvClosedLoopControl] -> Terminator16/1  "LongCtrl_axvClosedLoopControl"
  [PI_NetEngTorqInc] -> Terminator6/1  "LongCtrl_PI_NetEngTorqInc"
  [VlcInternalAcc] -> VlcInternalAcc/1  "LongCtrl_VlcInternalAcc"
  [SwDC_7] -> Terminator32/1  "LongCtrl_Sw2DC7"
  [SwDC_3] -> Terminator28/1  "LongCtrl_Sw2DC3"
  [axvTracActMean] -> Terminator19/1  "LongCtrl_axvTracActMean"
  [FF_NetEngTorq] -> Terminator7/1  "LongCtrl_FF_NetEngTorq"
  [SwEC_3] -> Terminator36/1  "LongCtrl_Sw2EC3"
  [DCEnable] -> Terminator11/1  "LongCtrl_DCEnable"
  [SwDC_1] -> Terminator26/1  "LongCtrl_Sw2DC1"
  [SwEC_4] -> Terminator29/1  "LongCtrl_Sw2EC4"
  [Tr_Ratio] -> Terminator14/1  "LongCtrl_Tr_Ratio"
  [ECEnable] -> Terminator10/1  "LongCtrl_ECEnable"
  [ACC_DecelReqValue] -> ACC_Decel_ReqValue/1  "LongCtrl_ACC_Decel_ReqValue"
  [axvTracMin] -> Terminator13/1  "LongCtrl_axvTracMin"
  [SwEC_5] -> Terminator30/1  "LongCtrl_Sw2EC5"
  [SwEC_2] -> Terminator35/1  "LongCtrl_Sw2EC2"
  [ACC_EngTorqReq] -> ACC_EngTrqReq/1  "LongCtrl_ACC_EngTrqReq"
  [SwDC_6] -> Terminator23/1  "LongCtrl_Sw2DC6"
  [PI_NetEngTorq] -> Terminator5/1  "LongCtrl_PI_NetEngTorq"
  [axvModelResidual] -> Terminator18/1  "LongCtrl_axvModelResidual"
  [SwEC_1] -> Terminator34/1  "LongCtrl_Sw2EC1"
  [ACC_EngTorqReqActive] -> ACC_EngTrqReqActive/1  "LongCtrl_ACC_EngTrqReqActive"
  [SwDC_2] -> Terminator27/1  "LongCtrl_Sw2DC2"
  Compare To Constant8/1 -> Signal Copy6/1
  VehicleStandstill/1 -> Compare To Constant8/1
  SHIFT_INPROGRESS/1 -> Signal Copy8/1
  Subsystem/1(ACCModeSts) -> Signal Copy14/1
  NetEngTrq_G/1 -> Signal Copy9/1
  NoBrakeForce/1 -> Signal Copy5/1
  Signal Copy/1 -> [VehSts_axvRoadSlope]  "LongCtrl_axvRoadSlopeMs2"
  ACC_DecelToStopReq/1 -> Signal Copy22/1
  ACC_axvCvAim/1 -> Signal Copy16/1
  Gain1/1 -> [VehSts_VxvRef_kmh]
  CURRENT_GEAR/1 -> Signal Copy7/1
  EngTqMaxActSpd/1 -> Signal Copy12/1
  MinMax1/1 -> Signal Copy10/1
  ACC_DecelerateJerk/1 -> Signal Copy19/1
  EngSpd/1 -> Signal Copy13/1
  MaxEngTorqNorm/1 -> MinMax1/2
  vxvRefMs/1 -> Signal Copy1/1
  ACC_DrvOFF_Req/1 -> Signal Copy15/1
  Product/1 -> Trigonometric Function/1
  ACC_AccelerateJerk/1 -> Signal Copy20/1
  ACC_axv_ComfortBandUpperValue/1 -> Signal Copy18/1
  ACC_axv_ComfortBandLowerValue/1 -> Signal Copy17/1
  Constant/1 -> MinMax1/1
  AxRefDt/1 -> Signal Copy4/1
  EngTqMinAct/1 -> Signal Copy11/1
  tCycleVLC/1 -> Signal Copy23/1
  [tCycleVLC] -> VlcInternalAccCalc/11(tCycleVLC)
  [tCycleVLC] -> PI_Control/16(tCycle)
  [tCycleVLC] -> EC/16(tCycle)
  [tCycleVLC] -> DC/5(tCycle)
  axvRoadSlopeMs2/1 -> Signal Copy/1
  Signal Copy1/1 -> [VehSts_VxvRef_ms], Gain1/1  "LongCtrl_vxvRefMs"
  Signal Copy2/1 -> [AxRef_ms2]  "Longctrl_VIE_axRefMs2"
  Signal Copy3/1 -> Terminator48/1  "Longctrl_VIE_alpSideSlipAngle"
  Signal Copy4/1 -> [VehSts_AxRefDt]  "Longctrl_VIE_AxRefDt"
  Signal Copy5/1 -> [CAN_NoBrakeForce]  "Longctrl_NoBrakeForce"
  Signal Copy6/1 -> [ACCSts_VehStandstill]  "Longctrl_VehicleStandStill"
  Signal Copy7/1 -> Goto/1  "Longctrl_CurrentGear"
  Signal Copy8/1 -> [CAN_ShiftInProgress]  "Longctrl_ShiftinProgress"
  Signal Copy9/1 -> [CAN_NetEngTrq]  "Longctrl_NetEngTrq"
  Signal Copy10/1 -> [CAN_MaxEngTrq]  "Longctrl_NetEngTorqNorm"
  Signal Copy11/1 -> [CAN_EngTqMinAct]  "Longctrl_EngTqMinAct"
  Signal Copy12/1 -> Goto8/1  "Longctrl_EngTqMaxActSpd"
  Signal Copy13/1 -> [CAN_EngSpd]  "Longctrl_EngSpd"
  Signal Copy14/1 -> [ACCSts_ACCModeSts]  "Longctrl_ACCSts"
  Signal Copy15/1 -> [ACCSts_DriveOffReq]  "Longctrl_ACC_DrvOFF_Req"
  Signal Copy16/1 -> [ACC_axvCvAim]  "Longctrl_ACC_axvCvAim"
  Signal Copy17/1 -> [ACC_axvComfortBandLowerValue]  "Longctrl_ACC_axv_ComfortBandLowerValue"
  Signal Copy18/1 -> [ACC_axvComfortBandUpperValue]  "Longctrl_ACC_axv_ComfortBandUpperValue"
  Signal Copy19/1 -> [ACC_LowerJerk]  "Longctrl_ACC_DecelerateJerk"
  Signal Copy20/1 -> [ACC_UpperJerk]  "Longctrl_ACC_AccelerateJerk"
  ACC_BrakePrefer/1 -> Signal Copy21/1
  Signal Copy21/1 -> [ACC_BrakePrefer]  "Longctrl_ACC_BrakePrefer"
  Signal Copy22/1 -> [ACC_DecelToStopReq]  "Longctrl_ACC_DecelToStopReq"
  Signal Copy23/1 -> [tCycleVLC]  "Longctrl_tCycleVLC"
  Signal Copy25/1 -> [DriveOffConditonFulfilled]  "LongCtrl_VLC_DriveOffConditonFulfilled"
  DriveOffConditonFulfilled/1 -> Signal Copy25/1
  FLWheelDriveDirection/1 -> Signal Copy24/1
  Signal Copy24/1 -> [FLWheelDriveDirection]  "LongCtrl_FLWheelDriveDirection"
  Signal Copy26/1 -> [FRWheelDriveDirection]  "LongCtrl_FRWheelDriveDirection"
  FRWheelDriveDirection/1 -> Signal Copy26/1
  RRWheelDriveDirection/1 -> Signal Copy28/1
  Signal Copy28/1 -> [RRWheelDriveDirection]  "LongCtrl_RRWheelDriveDirection"
  RLWheelDriveDirection/1 -> Signal Copy27/1
  Signal Copy27/1 -> [RLWheelDriveDirection]  "LongCtrl_RLWheelDriveDirection"
  [FLWheelDriveDirection] -> SlidJudge/1(FLWheelDriveDirection)
  [FRWheelDriveDirection] -> SlidJudge/2(FRWheelDriveDirection)
  [RLWheelDriveDirection] -> SlidJudge/3(RLWheelDriveDirection)
  [RRWheelDriveDirection] -> SlidJudge/4(RRWheelDriveDirection)
  [VehSts_axvRoadSlope] -> SlidJudge/5(LM_axvRoadSlopeMs2)
  [ACCSts_ACCModeSts] -> SlidJudge/6(ACCModeSts)
  [VehSts_VxvRef_ms] -> SlidJudge/7(vxvRef_ms)
  [Fz] -> SlidJudge/8(Fz)
  [CAN_NetEngTrq] -> SlidJudge/9(NetEngTrq)
  [CAN_MaxEngTrq] -> SlidJudge/10(MaxEngTrq)
  [Tr_Ratio] -> SlidJudge/11(Tr_Ratio)
  SlidJudge/1(SlideFlag) -> [SlideFlag]
  SlidJudge/2(ForwardFlag) -> [ForwardFlag]
  [SlideFlag] -> VLC_control_sts/7(SlideFlag)
  [ForwardFlag] -> VLC_control_sts/8(ForwardFlag)
  [DriveOffConditonFulfilled] -> VLC_control_sts/9(DriveOffConditonFulfilled)
  VLC_control_sts/5(VLCState) -> [VLCState]
  VLC_control_sts/6(tECDC) -> [tECDC]
  [tEC] -> Terminator4/1  "LongCtrl_tEC"
  [tECDC] -> Terminator1/1  "LongCtrl_tECDC"
  [VLCState] -> Terminator3/1  "LongCtrl_VLCState"
  [VLCState] -> DC/6(VLCState)
  [tECDC] -> EC/18(tECDC)
  [VLCState] -> EC/17(VLCState)

== system PvtSubSys_LONC/VLC/Vlc/DC ==
  DC_enable : Inport
  VlcAxTar : Inport  Port=2
  ACCmode : Inport  Port=3
  axvRoadSlopeMs2 : Inport  Port=4
  tCycle : Inport  Port=5
  VLCState : Inport  Port=6
  1-D Lookup Table : Lookup_n-D  NumberOfTableDimensions=1  BreakpointsForDimension1=P_LongCtrl_VLCaccelMinHoldXAxis  Table=P_LongCtrl_VLCaccelMinHoldYAxis  ExtrapMethod=Clip  UseLastTableValue=on  InternalRulePriority=Speed  OutDataTypeStr=single  RndMeth=Simplest  InputSameDT=on
  1-D Lookup Table1 : Lookup_n-D  NumberOfTableDimensions=1  BreakpointsForDimension1=P_LongCtrl_VLCjerkHoldXAxis  Table=P_LongCtrl_VLCjerkHoldYAxis  ExtrapMethod=Clip  UseLastTableValue=on  InternalRulePriority=Speed  OutDataTypeStr=single  RndMeth=Simplest  InputSameDT=on
  1-D Lookup Table2 : Lookup_n-D  NumberOfTableDimensions=1  BreakpointsForDimension1=P_LongCtrl_VLCaccelMinSlidHoldXAxis  Table=P_LongCtrl_VLCaccelMinSlidHoldYAxis  ExtrapMethod=Clip  InternalRulePriority=Speed  OutDataTypeStr=single  RndMeth=Simplest  InputSameDT=on
  1-D Lookup Table3 : Lookup_n-D  NumberOfTableDimensions=1  BreakpointsForDimension1=P_LongCtrl_VLCjerkSlidHoldXAxis  Table=P_LongCtrl_VLCjerkSlidHoldYAxis  ExtrapMethod=Clip  InternalRulePriority=Speed  OutDataTypeStr=single  RndMeth=Simplest  InputSameDT=on
  Logical Operator : Logic  Operator=OR  AllPortsSameDT=off  OutDataTypeStr=boolean
  Product1 : Product  RndMeth=Zero
  StandstillAccel2 : Stateflow chart  TreatAsAtomicUnit=on
      settings: PortSchema="{\"entries\":[{\"content\":{\"sides\":[{\"content\":{\"connectorIds\":[\"In1\",\"In2\",\"In7\",\"In8\",\"In3\",\"In4\",\"In5\",\"In6\"]},\"type\":\"ConnectorPlacement.EquallySpacedRectSide\",\"uuid\":\"10b5f078-7c95-4293-9ebe-1ebe87b8d3bb\"},{\"content\":{\"connectorIds\":[\"Out1\",\"Out2\"],\"side\":\"RIGHT\"},\"type\":\"ConnectorPlacement.EquallySpacedRectSide\",\"uuid\":\"a3eaf481-4607-4852-a8c0-60ae523e0874\"},{\"content\":{\"connectorIds\":[],\"side\":\"TOP\"},\"type\":\"ConnectorPlacement.EquallySpacedRectSide\",\"uuid\":\"24bfa6d2-2a60-4c58-bbb2-05df9b741c46\"},{\"content\":{\"connectorIds\":[],\"side\":\"HIDDEN\"},\"type\":\"ConnectorPlacement.EquallySpacedRectSide\",\"uuid\":\"641254b3-2cbc-43f7-a318-5e8a6a05f81c\"}]},\"type\":\"ConnectorPlacement.EquallySpacedConnector\",\"uuid\":\"ac8ab8d9-8adb-4650-a590-6d6465a6fba2\"}],\"packageUris\":[\"http://schema.mathworks.com/mf0/Connector/R2020b\"],\"version\":\"1.0\"}"
  Tapped Delay : simulink/Discrete/Tapped Delay  vinit=0.0  samptime=-1  NumDelays=1  DelayOrder=Newest  includeCurrent=on
  ACC_Decel_Req : Outport
  ACC_Decel_ReqValue : Outport  Port=2
  wires:
  1-D Lookup Table1/1 -> StandstillAccel2/4(jerkHold)  "LongCtrl_jerkHold"
  1-D Lookup Table/1 -> StandstillAccel2/3(accelHoldMin)  "LongCtrl_accelHoldMin"
  StandstillAccel2/2(decelReq) -> ACC_Decel_ReqValue/1
  ACCmode/1 -> Tapped Delay/1
  VlcAxTar/1 -> Product1/2
  DC_enable/1 -> Logical Operator/1, Product1/1
  Product1/1 -> StandstillAccel2/1(VlcAxTar)
  Tapped Delay/1 -> StandstillAccel2/2(ACCmode)
  StandstillAccel2/1(decelReqActive) -> Logical Operator/2
  Logical Operator/1 -> ACC_Decel_Req/1
  tCycle/1 -> StandstillAccel2/5(tCycle)
  1-D Lookup Table3/1 -> StandstillAccel2/8(jerkSlidHold)  "LongCtrl_jerkSlidHold"
  axvRoadSlopeMs2/1 -> 1-D Lookup Table2/1, 1-D Lookup Table3/1, 1-D Lookup Table/1, 1-D Lookup Table1/1
  1-D Lookup Table2/1 -> StandstillAccel2/7(accelSlidHold)  "LongCtrl_accelSlidHold"
  VLCState/1 -> StandstillAccel2/6(VLCState)

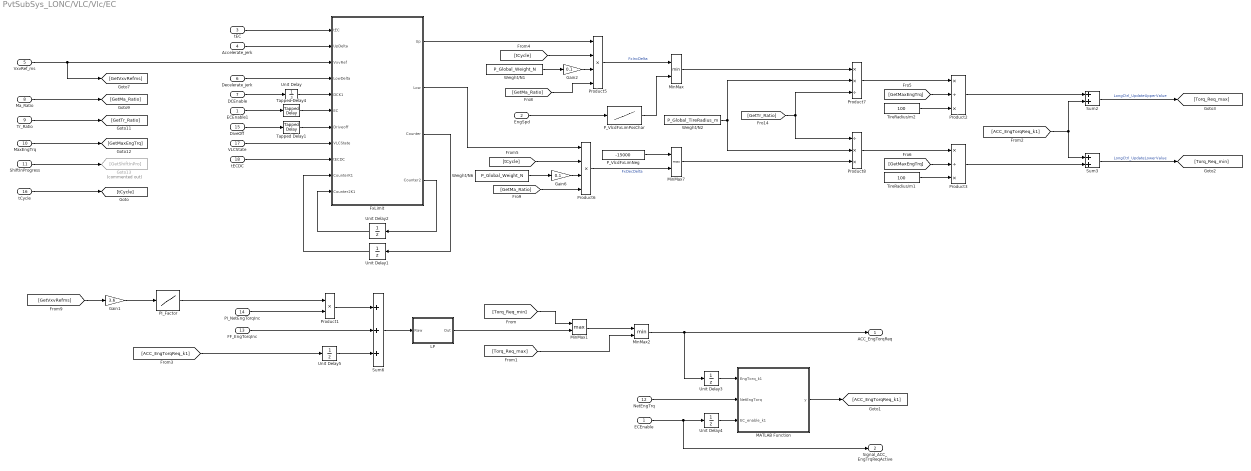
== system PvtSubSys_LONC/VLC/Vlc/EC ==
  ECEnable : Inport
  EngSpd : Inport  Port=2
  tEC : Inport  Port=3
  Accelerate_jerk : Inport  Port=4
  VxvRef_ms : Inport  Port=5
  Decelerate_jerk : Inport  Port=6
  DCEnable : Inport  Port=7
  Ma_Ratio : Inport  Port=8
  Tr_Ratio : Inport  Port=9
  MaxEngTrq : Inport  Port=10
  ShiftInProgress : Inport  Port=11
  NetEngTrq : Inport  Port=12
  FF_EngTorqInc : Inport  Port=13
  PI_NetEngTorqInc : Inport  Port=14
  DiveOff : Inport  Port=15  OutDataTypeStr=boolean
  tCycle : Inport  Port=16
  VLCState : Inport  Port=17
  tECDC : Inport  Port=18
  ECEnable1 : InportShadow
  FxLimit : MATLAB Function  TreatAsAtomicUnit=on
  Gain1 : Gain  Gain=3.6
  Gain2 : Gain  Gain=0.1
  Gain6 : Gain  Gain=0.1
  Goto13 : Goto  Commented=on  GotoTag=GetShiftInPro
  LP : Subsystem
  MATLAB Function : MATLAB Function  TreatAsAtomicUnit=on
  MinMax : MinMax  Inputs=2
  MinMax1 : MinMax  Function=max  Inputs=2
  MinMax2 : MinMax  Inputs=2
  MinMax7 : MinMax  Function=max  Inputs=2
  "PI_Factor " : Lookup_n-D  NumberOfTableDimensions=1  BreakpointsForDimension1=P_LongCtrl_VLCvelCharCoefPIXAxis  Table=P_LongCtrl_VLCcoefPIYAxis  ExtrapMethod=Clip  UseLastTableValue=on  RndMeth=Simplest  InputSameDT=on
  P_VlcdFxLimNeg : Constant  Value=-15000  OutDataTypeStr=single
  "P_VlcdFxLimPosChar " : Lookup_n-D  NumberOfTableDimensions=1  BreakpointsForDimension1=[500,1000,1100]  Table=[1500,3000,10000]  ExtrapMethod=Clip  UseLastTableValue=on  RndMeth=Simplest  InputSameDT=on
  Product1 : Product  RndMeth=Zero
  Product2 : Product  Inputs=*/*  RndMeth=Zero
  Product3 : Product  Inputs=*/*  RndMeth=Zero
  Product5 : Product  Inputs=4  RndMeth=Zero
  Product6 : Product  Inputs=4  RndMeth=Zero
  Product7 : Product  Inputs=**/  RndMeth=Zero
  Product8 : Product  Inputs=/**  RndMeth=Zero
  Sum2 : Sum
  Sum3 : Sum
  Sum6 : Sum  Inputs=+++
  Tapped Delay1 : simulink/Discrete/Tapped Delay  vinit=0.0  samptime=-1  NumDelays=1  DelayOrder=Newest  includeCurrent=on
  Tapped Delay4 : simulink/Discrete/Tapped Delay  vinit=0.0  samptime=-1  NumDelays=1  DelayOrder=Newest  includeCurrent=on
  TireRadius/m1 : Constant  Value=100  OutDataTypeStr=single
  TireRadius/m2 : Constant  Value=100  OutDataTypeStr=single
  Unit Delay{,3..5} (4 alike) : UnitDelay  SampleTime=-1  HasFrameUpgradeWarning=on
  Unit Delay1 : UnitDelay  InitialCondition=single(0)  SampleTime=-1  HasFrameUpgradeWarning=on
  Unit Delay2 : UnitDelay  InitialCondition=single(0)  SampleTime=-1  HasFrameUpgradeWarning=on
  Weight/N1 : Constant  Value=P_Global_Weight_N  OutDataTypeStr=single
  Weight/N2 : Constant  Value=P_Global_TireRadius_m  OutDataTypeStr=single
  Weight/N6 : Constant  Value=P_Global_Weight_N  OutDataTypeStr=single
  ACC_EngTorqReq : Outport
  Signal_ACC_EngTrqReqActive : Outport  Port=2
  wires:
  Unit Delay2/1 -> FxLimit/11(Counter2K1)
  FxLimit/4(Counter2) -> Unit Delay2/1
  Unit Delay1/1 -> FxLimit/10(CounterK1)
  NetEngTrq/1 -> MATLAB Function/2(NetEngTorq)
  [Torq_Req_max] -> MinMax2/2
  MinMax1/1 -> MinMax2/1
  [Torq_Req_min] -> MinMax1/1
  LP/1(Out) -> MinMax1/2
  Sum2/1 -> [Torq_Req_max]  "LongCtrl_UpdateUpperValue"
  [ACC_EngTorqReq_k1] -> Sum2/2, Sum3/1
  Product2/1 -> Sum2/1
  Sum3/1 -> [Torq_Req_min]  "LongCtrl_UpdateLowerValue"
  Product3/1 -> Sum3/2
  DiveOff/1 -> Tapped Delay1/1
  Tapped Delay4/1 -> FxLimit/6(EC)
  Tapped Delay1/1 -> FxLimit/7(Driveoff)
  Unit Delay/1 -> FxLimit/5(DCK1)
  MaxEngTrq/1 -> [GetMaxEngTrq]
  ShiftInProgress/1 -> Goto13/1
  Tr_Ratio/1 -> [GetTr_Ratio]
  Ma_Ratio/1 -> [GetMa_Ratio]
  Unit Delay5/1 -> Sum6/3
  [ACC_EngTorqReq_k1] -> Unit Delay5/1
  FF_EngTorqInc/1 -> Sum6/2
  Gain1/1 -> "PI_Factor "/1
  [GetVxvRefms] -> Gain1/1
  MinMax2/1 -> ACC_EngTorqReq/1, Unit Delay3/1
  VxvRef_ms/1 -> FxLimit/3(VxvRef), [GetVxvRefms]
  Sum6/1 -> LP/1(Raw)
  ECEnable1/1 -> Tapped Delay4/1
  FxLimit/3(Counter) -> Unit Delay1/1
  DCEnable/1 -> Unit Delay/1
  Product8/1 -> Product3/1
  [GetMaxEngTrq] -> Product3/2
  TireRadius/m1/1 -> Product3/3
  Product7/1 -> Product2/1
  [GetMaxEngTrq] -> Product2/2
  TireRadius/m2/1 -> Product2/3
  FxLimit/2(Low) -> Product6/1
  FxLimit/1(Up) -> Product5/1
  tEC/1 -> FxLimit/1(tEC)
  MinMax7/1 -> Product8/3
  [GetTr_Ratio] -> Product8/1, Product7/3
  Weight/N2/1 -> Product8/2, Product7/2
  MinMax/1 -> Product7/1
  [GetMa_Ratio] -> Product6/4
  Gain6/1 -> Product6/3
  Weight/N6/1 -> Gain6/1
  [tCycle] -> Product6/2
  Decelerate_jerk/1 -> FxLimit/4(LowDelta)
  [GetMa_Ratio] -> Product5/4
  P_VlcdFxLimNeg/1 -> MinMax7/1
  Product6/1 -> MinMax7/2  "FxDecDelta"
  "P_VlcdFxLimPosChar "/1 -> MinMax/2
  EngSpd/1 -> "P_VlcdFxLimPosChar "/1
  Product5/1 -> MinMax/1  "FxIncDelta"
  Gain2/1 -> Product5/3
  Weight/N1/1 -> Gain2/1
  [tCycle] -> Product5/2
  Accelerate_jerk/1 -> FxLimit/2(UpDelta)
  Unit Delay4/1 -> MATLAB Function/3(EC_enable_k1)
  ECEnable/1 -> Unit Delay4/1, Signal_ACC_EngTrqReqActive/1
  Product1/1 -> Sum6/1
  "PI_Factor "/1 -> Product1/1
  PI_NetEngTorqInc/1 -> Product1/2
  MATLAB Function/1(y) -> [ACC_EngTorqReq_k1]
  Unit Delay3/1 -> MATLAB Function/1(EngTorq_k1)
  tCycle/1 -> [tCycle]
  VLCState/1 -> FxLimit/8(VLCState)
  tECDC/1 -> FxLimit/9(tECDC)

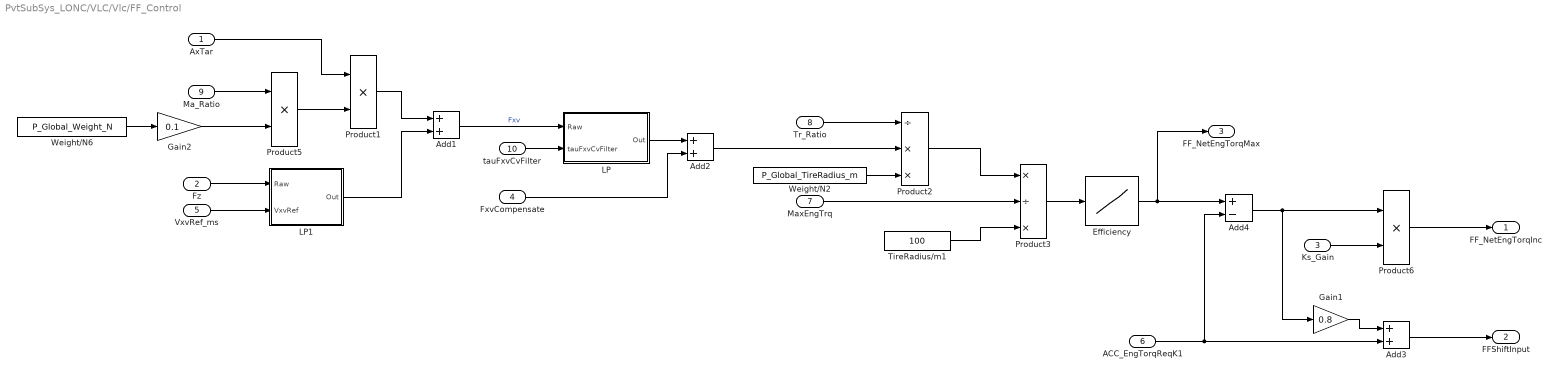
== system PvtSubSys_LONC/VLC/Vlc/FF_Control ==
  AxTar : Inport  OutDataTypeStr=single
  Fz : Inport  Port=2  OutDataTypeStr=single
  Ks_Gain : Inport  Port=3  OutDataTypeStr=single
  FxvCompensate : Inport  Port=4  OutDataTypeStr=single
  VxvRef_ms : Inport  Port=5  OutDataTypeStr=single
  ACC_EngTorqReqK1 : Inport  Port=6  OutDataTypeStr=single
  MaxEngTrq : Inport  Port=7  OutDataTypeStr=single
  Tr_Ratio : Inport  Port=8  OutDataTypeStr=single
  Ma_Ratio : Inport  Port=9  OutDataTypeStr=single
  tauFxvCvFilter : Inport  Port=10  OutDataTypeStr=single
  Add1 : Sum
  Add2 : Sum
  Add3 : Sum
  Add4 : Sum  Inputs=+-
  Efficiency : Lookup_n-D  NumberOfTableDimensions=1  BreakpointsForDimension1=P_LongCtrl_VLCtorqCharEngInverseEfficientXAxis  Table=P_LongCtrl_VLCengInverseEfficientYAxis  ExtrapMethod=Clip  UseLastTableValue=on  RndMeth=Simplest  InputSameDT=on
  Gain1 : Gain  Gain=0.8
  Gain2 : Gain  Gain=0.1
  LP : Subsystem
  LP1 : Subsystem
  Product1 : Product  RndMeth=Zero
  Product2 : Product  Inputs=/**  RndMeth=Zero
  Product3 : Product  Inputs=*/*  RndMeth=Zero
  Product5 : Product  Inputs=**  RndMeth=Zero
  Product6 : Product  RndMeth=Zero
  TireRadius/m1 : Constant  Value=100  OutDataTypeStr=single
  Weight/N2 : Constant  Value=P_Global_TireRadius_m
  Weight/N6 : Constant  Value=P_Global_Weight_N
  FF_NetEngTorqInc : Outport  OutDataTypeStr=single
  FFShiftInput : Outport  Port=2  OutDataTypeStr=single
  FF_NetEngTorqMax : Outport  Port=3  OutDataTypeStr=single
  wires:
  tauFxvCvFilter/1 -> LP/2(tauFxvCvFilter)
  VxvRef_ms/1 -> LP1/2(VxvRef)
  LP1/1(Out) -> Add1/2
  Tr_Ratio/1 -> Product2/1
  Add3/1 -> FFShiftInput/1
  Gain1/1 -> Add3/1
  ACC_EngTorqReqK1/1 -> Add4/2, Add3/2
  FxvCompensate/1 -> Add2/2
  LP/1(Out) -> Add2/1
  Add4/1 -> Gain1/1, Product6/1
  Add2/1 -> Product2/2
  Add1/1 -> LP/1(Raw)  "Fxv"
  Product6/1 -> FF_NetEngTorqInc/1
  Ks_Gain/1 -> Product6/2
  AxTar/1 -> Product1/1
  Efficiency/1 -> Add4/1, FF_NetEngTorqMax/1
  Weight/N2/1 -> Product2/3
  Product1/1 -> Add1/1
  Fz/1 -> LP1/1(Raw)
  Product3/1 -> Efficiency/1
  Product2/1 -> Product3/1
  MaxEngTrq/1 -> Product3/2
  TireRadius/m1/1 -> Product3/3
  Weight/N6/1 -> Gain2/1
  Gain2/1 -> Product5/2
  Product5/1 -> Product1/2
  Ma_Ratio/1 -> Product5/1

== system PvtSubSys_LONC/VLC/Vlc/LP ==
  Raw : Inport
  Constant2 : Constant  Value=0.02  OutDataTypeStr=single
  FilterTime1 : Constant  Value=0.1  OutDataTypeStr=single
  Product2 : Product  Inputs=*/  RndMeth=Zero
  Product6 : Product  RndMeth=Zero
  Sum6 : Sum  Inputs=+-  OutDataTypeStr=single
  Sum7 : Sum  OutDataTypeStr=single
  Unit Delay : UnitDelay  SampleTime=-1  HasFrameUpgradeWarning=on
  Out : Outport
  wires:
  Raw/1 -> Sum6/1
  Product6/1 -> Sum7/1
  Product2/1 -> Product6/1
  Sum6/1 -> Product6/2
  FilterTime1/1 -> Product2/2
  Constant2/1 -> Product2/1
  Unit Delay/1 -> Sum7/2, Sum6/2
  Sum7/1 -> Out/1, Unit Delay/1

== system PvtSubSys_LONC/VLC/Vlc/LP1 ==
  Raw : Inport
  Constant2 : Constant  Value=0.02  OutDataTypeStr=single
  FilterTime1 : Constant  Value=0.1  OutDataTypeStr=single
  Product2 : Product  Inputs=*/  RndMeth=Zero
  Product6 : Product  RndMeth=Zero
  Sum6 : Sum  Inputs=+-
  Sum7 : Sum
  Unit Delay : UnitDelay  SampleTime=-1  HasFrameUpgradeWarning=on
  Out : Outport
  wires:
  Raw/1 -> Sum6/1
  Product6/1 -> Sum7/1
  Product2/1 -> Product6/1
  Sum6/1 -> Product6/2
  FilterTime1/1 -> Product2/2
  Constant2/1 -> Product2/1
  Unit Delay/1 -> Sum6/2, Sum7/2
  Sum7/1 -> Unit Delay/1, Out/1
